simulink model "p2_rcrc_sim"  (R2024a)
settings: Solver=ode3  StartTime=0.0  StopTime=0.1  FixedStep=Ts  MaxStep=1/20e3  RelTol=1e-3
PostLoadFcn:
  | try
  | if isempty(which('ZHAWcbfcn'));
  | callback_fid07124=fopen('ZHAWcbfcn.m','w');
  | [~]=fprintf(callback_fid07124,'%s',get_param([bdroot,'/ Setup SLDRT'],'ClipboardFcn'));
  | [~]=fclose(callback_fid07124);
  | setpref('ZHAW_SLDRT_lib','cb_fcn',which('ZHAWcbfcn'))
  | clear callback_fid07124
  | end
  | catch
  | clear callback_fid07124
  | end
  | Ts=eval(get_param([bdroot,'/ Setup SLDRT'],'Ts'));
InitFcn:
  | Ts=eval(get_param([bdroot,'/ Setup SLDRT'],'Ts'));
values from neighbouring files (symbols this model uses):
  a = R1*R2*C1*C2    (= 4.879681e-06)    [p2_rcrc_p_ini.m]
  b = R1*C1 + R1*C2 + R2*C2    (= 0.006627)    [p2_rcrc_p_ini.m]
  C1 = 470e-9    (= 4.7e-07)    [p2_rcrc_p_ini.m]
  C2 = C1    (= 4.7e-07)    [p2_rcrc_p_ini.m]
  R1 = 4.7e3    (= 4700)    [p2_rcrc_p_ini.m]
  R2 = R1    (= 4700)    [p2_rcrc_p_ini.m]
libraries: sldrtlib x1
(part 2 of 2)

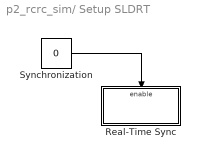
== system p2_rcrc_sim/ Setup SLDRT ==
  Real-Time Sync : Subsystem
  Synchronization : Constant  Value=0
  wires:
  Synchronization/1 -> Real-Time Sync/Enable

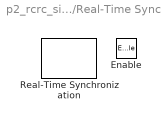
== system p2_rcrc_sim/ Setup SLDRT/Real-Time Sync ==
  Enable : EnablePort
  Real-Time Synchronization : sldrtlib/Real-Time Synchronization  SampleTime=Ts  MaxMissedTicks=inf  ShowMissedTicks=off  YieldWhenWaiting=off
